simulink model "eq_4khz"  (R2023a)
settings: Solver=VariableStepAuto  StartTime=0.0  StopTime=10.0  RelTol=1e-3
libraries: spspowerguiLib x1
settings Model: Creator=86198  LastModifiedBy=86198

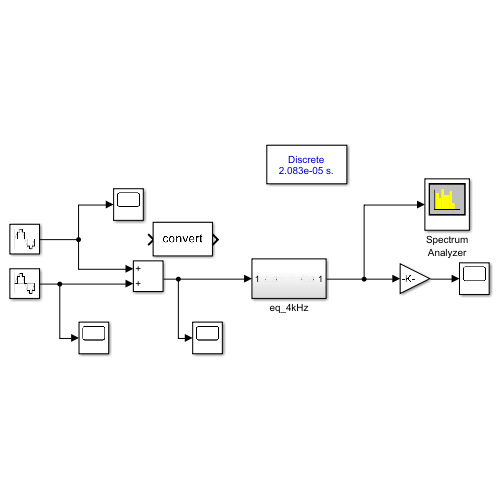
[thumbnail: Simulink's stored preview of the top-level diagram]
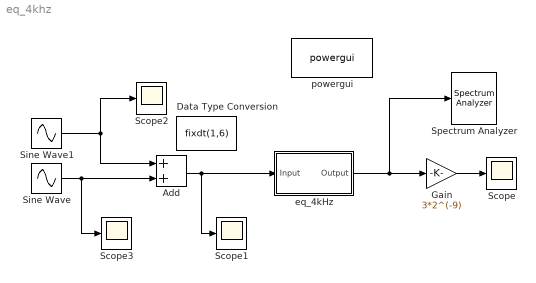
== system eq_4khz ==
  Add : Sum
  Data Type Conversion : DataTypeConversion  OutMin=[-1.5/1.1]  OutMax=[1.5/1.1]  OutDataTypeStr=fixdt(1,6)  SaturateOnIntegerOverflow=off  RndMeth=Floor
  Gain : Gain  Gain=3*2^(-9)
  Scope{,1..3} (4 alike) : Scope
  Sine Wave : Sin  Frequency=2*pi*4000  SampleTime=1/48000
  Sine Wave1 : Sin  Frequency=2*pi*1000  SampleTime=1/48000
  Spectrum Analyzer : SpectrumAnalyzer  WindowPosition=[320.000000,230.000000,800.000000,500.000000,]  ScopeFrameLocation=window  YLimits=[-190.60344926,114.94228451]  ColorLimits=[-20 80]  DefaultConfigurationName=spbscopes.SpectrumAnalyzerBlockCfg  IsFrequencyInputMode=0  FrequencyVectorPort=0  FrequencyVectorFromPort=0  FrequencyInputRBWPort=0  FrequencyInputRBWFromPort=0
  eq_4kHz : Subsystem  Tag=FilterWizardSubSystem
      settings: ErrorFcn=dspFilterRealizedInBasicElemsAlgLoopErrFcnCallback
  powergui : spspowerguiLib/powergui  Priority=1  SimulationMode=Discrete  SampleTime=1/48000  frequency=60  Iterations=50  frequencyindice=60  Pbase=100e6  ErrMax=1e-4  UnitsV=kV  UnitsW=MW  buscounter=0  FunctionMessages=off  echomessages=off  EnableUseOfTLC=off  CurrentSourceSwitches=off  DisableSnubberDevices=off  DisableRonSwitches=off  DisableVfSwitches=off  DisplayEquations=off  AutomaticDiscreteSolvers=off  SolverType=Tustin/Backward Euler (TBE)  Interpol=off  ExternalGateDelay=off  methode=off  Ts=100  x0status=blocks  SPID=on  SwTol=0  HookPort=off  NonlinearTolerance=1e-4  nMaxIteration=100  ContinueOnMaxIteration=off  RestoreLinks=warning  ResistiveCurrentMeasurement=off  Frange=[0:2:500]  Ylog=off  Xlog=on  ShowGrid=off  save=off  variable=ZData  structure=0  ZoomFFT=off  StartTime=0.0  cycles=1  DisplayStyle=1  fundamental=60  FreqAxis=off  MaxFrequency=1000  frequencyindicesteady=1  RmsSteady=1  display=off
  wires:
  Add/1 -> Scope1/1, eq_4kHz/1(Input)
  Sine Wave1/1 -> Add/1, Scope2/1
  Sine Wave/1 -> Add/2, Scope3/1
  Gain/1 -> Scope/1
  eq_4kHz/1(Output) -> Gain/1, Spectrum Analyzer/1

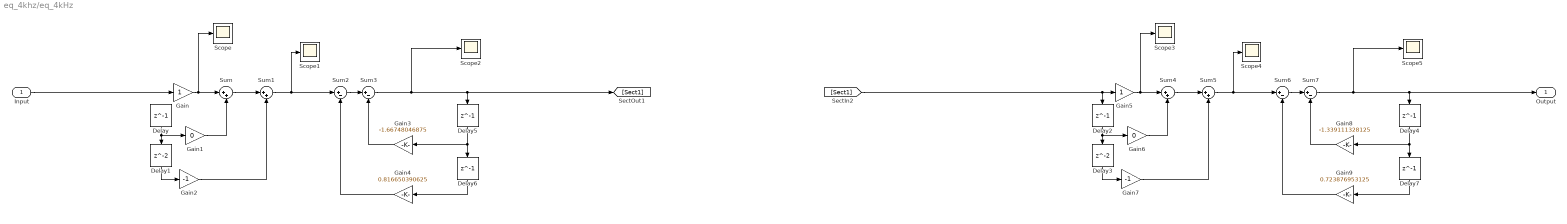
== system eq_4khz/eq_4kHz ==
  Input : Inport
  Delay{,2,4..7} (6 alike) : Delay  DelayLength=1
  Delay1 : Delay
  Delay3 : Delay
  Gain : Gain
  Gain1 : Gain  Gain=0
  Gain2 : Gain  Gain=-1
  Gain3 : Gain  Gain=-1.66748046875
  Gain4 : Gain  Gain=0.816650390625
  Gain5 : Gain
  Gain6 : Gain  Gain=0
  Gain7 : Gain  Gain=-1
  Gain8 : Gain  Gain=-1.339111328125
  Gain9 : Gain  Gain=0.723876953125
  Scope{,1..5} (6 alike) : Scope
  Sum{,1,4..5} (4 alike) : Sum  Inputs=|++
  Sum{2..3,6..7} (4 alike) : Sum  Inputs=|+-
  Output : Outport
  wires:
  Delay/1 -> Delay1/1, Gain1/1
  Sum2/1 -> Sum3/1
  Gain2/1 -> Sum1/2
  Gain1/1 -> Sum/2
  Sum1/1 -> Scope1/1, Sum2/1
  Sum3/1 -> Scope2/1, [Sect1], Delay5/1
  Delay6/1 -> Gain4/1
  Delay5/1 -> Delay6/1, Gain3/1
  Gain3/1 -> Sum3/2
  Gain4/1 -> Sum2/2
  Sum/1 -> Sum1/1
  Gain/1 -> Scope/1, Sum/1
  Delay1/1 -> Gain2/1
  Delay2/1 -> Delay3/1, Gain6/1
  Sum5/1 -> Scope4/1, Sum6/1
  Sum7/1 -> Scope5/1, Output/1, Delay4/1
  Gain8/1 -> Sum7/2
  Delay7/1 -> Gain9/1
  Gain7/1 -> Sum5/2
  Delay4/1 -> Delay7/1, Gain8/1
  Gain6/1 -> Sum4/2
  Gain5/1 -> Scope3/1, Sum4/1
  Gain9/1 -> Sum6/2
  Delay3/1 -> Gain7/1
  Sum6/1 -> Sum7/1
  Sum4/1 -> Sum5/1
  [Sect1] -> Gain5/1, Delay2/1
  Input/1 -> Gain/1
